simulink model "HVDCU_B12_thyristor"  (R2024a)
settings: Solver=VariableStepAuto  StartTime=0.0  StopTime=0.04  RelTol=1e-3
undefined symbols (not defined in the file or in its folder): D1, Delta
libraries: spsThyristorLib x12, spsVoltageMeasurementLib x10, spsCurrentMeasurementLib x1, spsSeriesRLCBranchLib x1, spsThreePhaseTransformerThreeWindingsLib x1, spsThreePhaseSourceLib x1, sps_lib x1
settings Model: Creator=E370_  LastModifiedBy=E370_

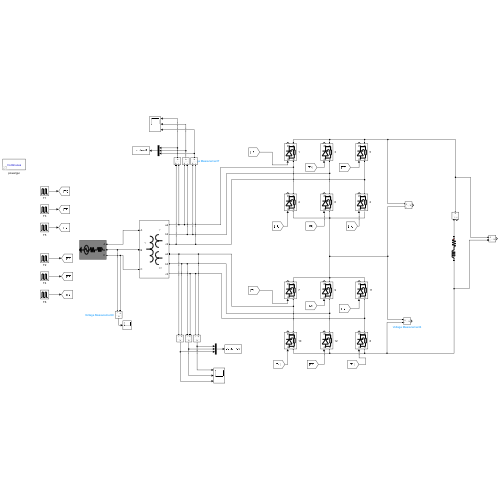
[thumbnail: Simulink's stored preview of the top-level diagram]
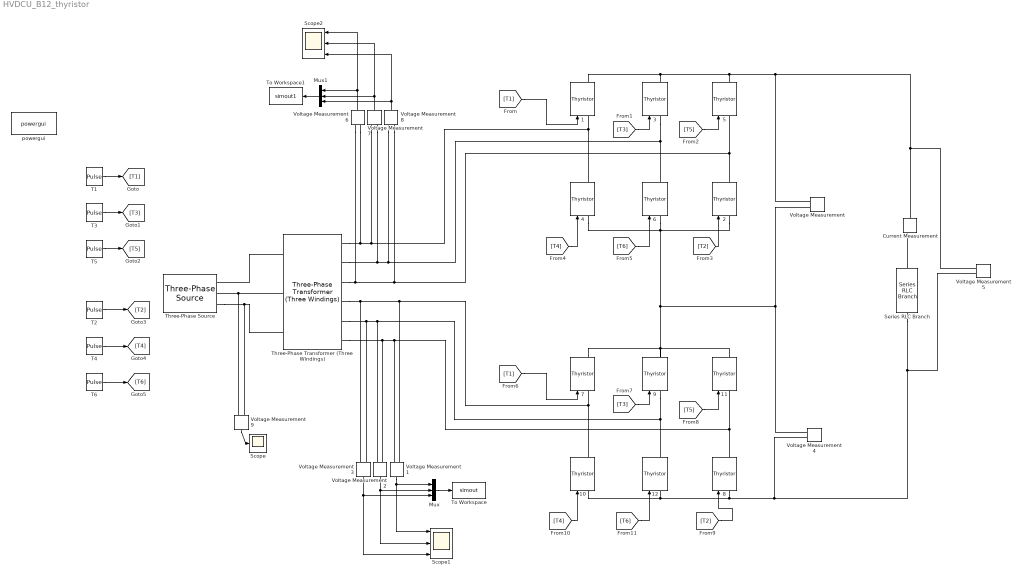
== system HVDCU_B12_thyristor ==
  {1..12} (12 alike) : spsThyristorLib/Thyristor  Ron=0.001  Lon=0  Vf=0.8  IC=0  Rs=500  Cs=250e-9  Measurements=on
  Current Measurement : spsCurrentMeasurementLib/Current Measurement  PhasorSimulation=off  OutputType=Complex  PSBequivalent=0
  Mux : Mux  Inputs=3
  Mux1 : Mux  Inputs=3
  Scope : Scope
  Scope1 : Scope  NumInputPorts=3
  Scope2 : Scope  NumInputPorts=3
  Series RLC Branch : spsSeriesRLCBranchLib/Series RLC Branch  LConnTagsString=__new0  RConnTagsString=__new0  BranchType=RL  Resistance=5000  Inductance=100e-3  SetiL0=off  InitialCurrent=0  Capacitance=1e-6  Setx0=off  InitialVoltage=0  Measurements=None
  T1 : DiscretePulseGenerator  PulseType=Time based  Period=0.02  PulseWidth=5  PhaseDelay=0.00334
  T2 : DiscretePulseGenerator  PulseType=Time based  Period=0.02  PulseWidth=5  PhaseDelay=0.00668
  T3 : DiscretePulseGenerator  PulseType=Time based  Period=0.02  PulseWidth=5  PhaseDelay=0.01
  T4 : DiscretePulseGenerator  PulseType=Time based  Period=0.02  PulseWidth=5  PhaseDelay=0.00334+0.01
  T5 : DiscretePulseGenerator  PulseType=Time based  Period=0.02  PulseWidth=5  PhaseDelay=0.01+0.00668
  T6 : DiscretePulseGenerator  PulseType=Time based  Period=0.02  PulseWidth=5
  Three-Phase Transformer (Three Windings) : spsThreePhaseTransformerThreeWindingsLib/Three-Phase Transformer (Three Windings)  Winding1Connection=Y  Winding2Connection=Y  Winding3Connection=Delta (D1)  CoreType=Three single-phase transformers  SetSaturation=off  Hysteresis=off  DataFile='hysteresis'  SetInitialFlux=off  Measurements=None  UNITS=pu  NominalPower=[ 250e6 , 50 ]  Winding1=[300 0.02 0]  Winding2=[100 0.02 0]  Winding3=[100 0.02 0]  Rm=500  Lm=500  L0=0.5  Saturation=[ 0,0 ; 0.0024,1.2 ; 1.0,1.52 ]  InitialFluxes=[0.8 -0.8 0.7]  BreakLoop=off  DiscreteSolver=Trapezoidal iterative  DataType=off  TransfoNumber=1
      settings: LibrarySourceBlock=|
      | sps_lib/Power Grid Elements/Three-Phase
      | Transformer
      | (Three Windings)
  Three-Phase Source : spsThreePhaseSourceLib/Three-Phase Source  InternalConnection=Yg  VoltagePhases=off  Voltage=100  PhaseAngle=0  Voltage_phases=[25e3 25e3 25e3]/sqrt(3)  PhaseAngles_phases=[0 -120 +120]  Frequency=50  NonIdealSource=on  SpecifyImpedance=off  Resistance=0.8929  Inductance=16.58e-3  ShortCircuitLevel=100e6  BaseVoltage=25e3  XRratio=7  BusType=swing  Pref=10e3  Qref=0  Prefabc=[10e3, 10e3, 10e3]  Qrefabc=[0, 0, 0]  Qmin=-inf  Qmax=inf
  To Workspace : ToWorkspace  VariableName=simout  SaveFormat=Timeseries  SampleTime=-1
  To Workspace1 : ToWorkspace  VariableName=simout1  SaveFormat=Timeseries  SampleTime=-1
  Voltage Measurement{,1..9} (10 alike) : spsVoltageMeasurementLib/Voltage Measurement  PhasorSimulation=off  OutputType=Complex  PSBequivalent=0
  powergui : sps_lib/powergui  Priority=1  SimulationMode=Continuous  SampleTime=50e-6  frequency=60  Iterations=50  frequencyindice=50  Pbase=100e6  ErrMax=1e-4  UnitsV=kV  UnitsW=MW  buscounter=0  FunctionMessages=off  echomessages=off  EnableUseOfTLC=off  CurrentSourceSwitches=off  DisableSnubberDevices=off  DisableRonSwitches=off  DisableVfSwitches=off  DisplayEquations=off  AutomaticDiscreteSolvers=off  SolverType=Tustin/Backward Euler (TBE)  Interpol=off  ExternalGateDelay=off  methode=off  Ts=100  x0status=blocks  SPID=on  SwTol=0  HookPort=off  NonlinearTolerance=1e-4  nMaxIteration=100  ContinueOnMaxIteration=off  RestoreLinks=warning  ResistiveCurrentMeasurement=off  Frange=[0:2:500]  Ylog=off  Xlog=on  ShowGrid=off  save=off  variable=ZData  structure=0  ZoomFFT=off  StartTime=0.0  cycles=1  DisplayStyle=1  fundamental=60  FreqAxis=off  MaxFrequency=1000  frequencyindicesteady=1  RmsSteady=1  display=off
  wires:
  Voltage Measurement1/1 -> Mux/1, Scope1/1
  Voltage Measurement2/1 -> Mux/2, Scope1/2
  [T6] -> 6/1
  [T4] -> 4/1
  [T5] -> 5/1
  [T1] -> 1/1
  T3/1 -> [T3]
  T5/1 -> [T5]
  T6/1 -> [T6]
  T1/1 -> [T1]
  Mux/1 -> To Workspace/1
  T4/1 -> [T4]
  T2/1 -> [T2]
  [T2] -> 2/1
  Voltage Measurement3/1 -> Mux/3, Scope1/3
  [T3] -> 3/1
  [T2] -> 8/1
  [T3] -> 9/1
  [T4] -> 10/1
  [T5] -> 11/1
  [T6] -> 12/1
  [T1] -> 7/1
  Voltage Measurement8/1 -> Mux1/3, Scope2/3
  Mux1/1 -> To Workspace1/1
  Voltage Measurement7/1 -> Mux1/2, Scope2/2
  Voltage Measurement6/1 -> Mux1/1, Scope2/1
  Voltage Measurement9/1 -> Scope/1
  connections:
  3/RConn1 -- Voltage Measurement5/LConn1 -- Current Measurement/LConn1 -- Voltage Measurement/LConn1 -- 5/RConn1 -- 1/RConn1
  3/LConn1 -- Voltage Measurement8/LConn1 -- Voltage Measurement7/LConn2 -- Three-Phase Transformer (Three Windings)/RConn2 -- 6/RConn1
  4/RConn1 -- Voltage Measurement6/LConn2 -- Three-Phase Transformer (Three Windings)/RConn1 -- Voltage Measurement7/LConn1 -- 1/LConn1
  2/RConn1 -- Voltage Measurement6/LConn1 -- Three-Phase Transformer (Three Windings)/RConn3 -- Voltage Measurement8/LConn2 -- 5/LConn1
  Three-Phase Transformer (Three Windings)/LConn2 -- Three-Phase Source/RConn2 -- Voltage Measurement9/LConn2
  Three-Phase Transformer (Three Windings)/LConn1 -- Three-Phase Source/RConn1
  Three-Phase Source/RConn3 -- Voltage Measurement9/LConn1 -- Three-Phase Transformer (Three Windings)/LConn3
  12/LConn1 -- Voltage Measurement5/LConn2 -- Series RLC Branch/RConn1 -- Voltage Measurement4/LConn2 -- 8/LConn1 -- 10/LConn1
  9/RConn1 -- Voltage Measurement4/LConn1 -- Voltage Measurement/LConn2 -- 2/LConn1 -- 4/LConn1 -- 6/LConn1 -- 11/RConn1 -- 7/RConn1
  10/RConn1 -- Voltage Measurement1/LConn1 -- Three-Phase Transformer (Three Windings)/RConn4 -- Voltage Measurement3/LConn2 -- 7/LConn1
  8/RConn1 -- Voltage Measurement1/LConn2 -- Voltage Measurement2/LConn1 -- Three-Phase Transformer (Three Windings)/RConn6 -- 11/LConn1
  9/LConn1 -- Voltage Measurement2/LConn2 -- Voltage Measurement3/LConn1 -- Three-Phase Transformer (Three Windings)/RConn5 -- 12/RConn1
  Series RLC Branch/LConn1 -- Current Measurement/RConn1
